simulink model "nmpc_sim"  (Simulink 8.8)
settings: Solver=ode45  StartTime=0.0  StopTime=20  RelTol=1e-3  EnableMultiTasking=on
InitFcn:
  | clear;close all;clc;
  | 
  | a=[-0.1832;558;118.45;9.6154e+03;...
  |     1.3712;5.1011e+03;641;426;6557;7.34;4484;0.016];
  | k=1;
  | x5d=50;
  | 
  | Ts=1e-4;
  | 
  | du=0.005;
StopFcn:
  | for i=1:4
  |     X(1:length(Measurements.signals(i).values(:,2)),i)=Measurements.signals(i).values(:,2);
  |     Xd(1:length(Measurements.signals(i).values(:,1)),i)=Measurements.signals(i).values(:,1);
  | end
  | 
  | U=Control.signals(2).values;
  | Ud=Control.signals(1).values;
  | 
  | Tnmpc=tnmpc.signals(1).values;
  | 
  | save exp_data X Xd U Ud Tnmpc;
values from neighbouring files (symbols this model uses):
  tnmpc = telapse/Ns    [nmpc_acado.m]
  ud = u(9)    [nmpc_acado.m]
undefined symbols (not defined in the file or in its folder): xd
settings Model: Creator=TIEUPHI  LastModifiedBy=trinhvv-admin
settings DataIOCC: SaveFormat=StructureWithTime  SignalLoggingSaveFormat=Dataset
settings DebuggingCC: UnderspecifiedInitializationDetection=Simplified  MergeDetectMultiDrivingBlocksExec=error  AllowSymbolicDim=off  StateNameClashWarn=none
settings HardwareCC: ProdBitPerPointer=64  ProdLargestAtomicFloat=Float  ProdIntDivRoundTo=Zero  ProdEndianess=LittleEndian  ProdHWDeviceType=Specified
settings GRTTargetCC: GeneratePreprocessorConditionals=Use local settings  CombineOutputUpdateFcns=on  GRTInterface=off

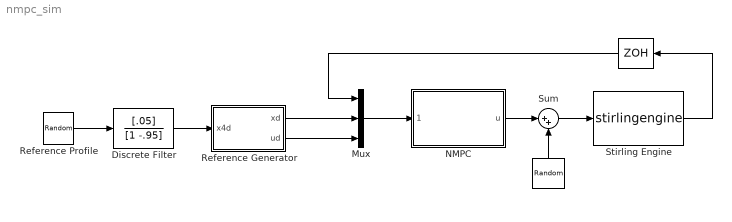
== system nmpc_sim ==
  "  " : ZeroOrderHold  SampleTime=Ts
  "   " : UniformRandomNumber  Minimum=-du  Maximum=du  Seed=1  SampleTime=Ts
  Discrete Filter : DiscreteFilter  Numerator=[.05]  Denominator=[1 -.95]  InitialStates=10.08*20  SampleTime=Ts
  Mux : Mux  Inputs=3
  NMPC : Subsystem
  Reference Generator : Subsystem
      mask init:
      | load ref_gen;
  Reference Profile : UniformRandomNumber  Minimum=7  Maximum=13  Seed=1234531  SampleTime=.5
  Stirling Engine : S-Function  InitFcn=try, set_param(gcb,'FunctionName','stirlingengine'), end  FunctionName=stirlingengine  Parameters=a,k,x5d  SFunctionModules=stirlingengine_wrapper  WizardData=DataTag0  SFunctionDeploymentMode=off  EnableBusSupport=off  mask(S-Function Builder){}
      mask help: Simulink:masks:SFunctionBuilder_MD
      mask init:
      | val = [[.9  0.75 0.75 1 1 .9 .9 1]',[1 1 0.75 0.75 .9 .9 1 .9]'];try , sys = get_param(gcb,'SfunBuilderFcnName');if isempty(sys), sys = get_param(gcb,'FunctionName'); end,catch, sys = get_param(gcb,'FunctionName'); end
      settings: CopyFcn=set_param(gcbh,'LinkStatus','none')  PreSaveFcn=try, set_param(gcb,'FunctionName','stirlingengine'), end  OpenFcn=sfunctionwizard(gcbh)
      mask Display: plot(val(:,1),val(:,2)),disp(sys), port_label('input',1,'u'), port_label('output',1,'y')
  Sum : Sum  Inputs=|++
  wires:
  Reference Generator/2(ud) -> Mux/3
  Reference Generator/1(xd) -> Mux/2
  Mux/1 -> NMPC/1(" ")
  Stirling Engine/1 -> "  "/1
  "  "/1 -> Mux/1
  Discrete Filter/1 -> Reference Generator/1(x4d)
  Reference Profile/1 -> Discrete Filter/1
  "   "/1 -> Sum/2
  NMPC/1(u) -> Sum/1
  Sum/1 -> Stirling Engine/1

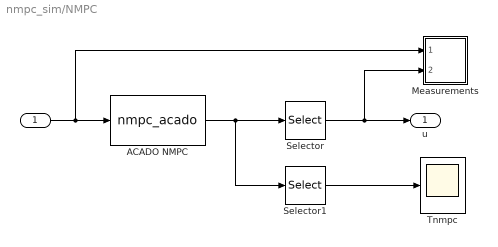
== system nmpc_sim/NMPC ==
  " " : Inport
  ACADO NMPC : MATLABFcn  MATLABFcn=nmpc_acado  OutputDimensions=2  OutputSignalType=real  SampleTime=Ts
  Measurements : Subsystem
  Selector : Selector  IndexOptions=Index vector (dialog)  Indices=1  OutputSizes=1
  Selector1 : Selector  IndexOptions=Index vector (dialog)  Indices=2  OutputSizes=1
  Tnmpc : Scope
  u : Outport
  wires:
  " "/1 -> Measurements/1(" "), ACADO NMPC/1
  ACADO NMPC/1 -> Selector1/1, Selector/1
  Selector/1 -> Measurements/2("   "), u/1
  Selector1/1 -> Tnmpc/1

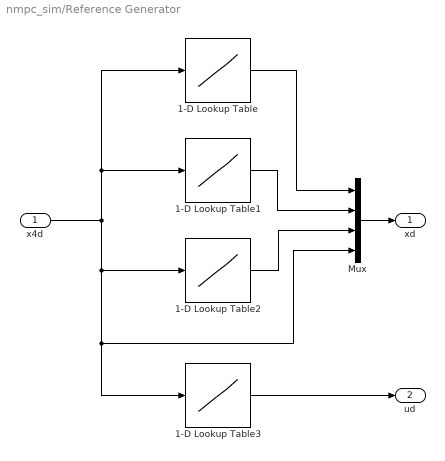
== system nmpc_sim/Reference Generator ==
  x4d : Inport
  1-D Lookup Table : Lookup_n-D  NumberOfTableDimensions=1  BreakpointsForDimension1=xd(:,4)  Table=xd(:,1)  RndMeth=Simplest  InputSameDT=on
  1-D Lookup Table1 : Lookup_n-D  NumberOfTableDimensions=1  BreakpointsForDimension1=xd(:,4)  Table=xd(:,2)  RndMeth=Simplest  InputSameDT=on
  1-D Lookup Table2 : Lookup_n-D  NumberOfTableDimensions=1  BreakpointsForDimension1=xd(:,4)  Table=xd(:,3)  RndMeth=Simplest  InputSameDT=on
  1-D Lookup Table3 : Lookup_n-D  NumberOfTableDimensions=1  BreakpointsForDimension1=xd(:,4)  Table=ud  RndMeth=Simplest  InputSameDT=on
  Mux : Mux
  xd : Outport
  ud : Outport  Port=2
  wires:
  x4d/1 -> Mux/4, 1-D Lookup Table3/1, 1-D Lookup Table2/1, 1-D Lookup Table1/1, 1-D Lookup Table/1
  Mux/1 -> xd/1
  1-D Lookup Table/1 -> Mux/1
  1-D Lookup Table1/1 -> Mux/2
  1-D Lookup Table2/1 -> Mux/3
  1-D Lookup Table3/1 -> ud/1

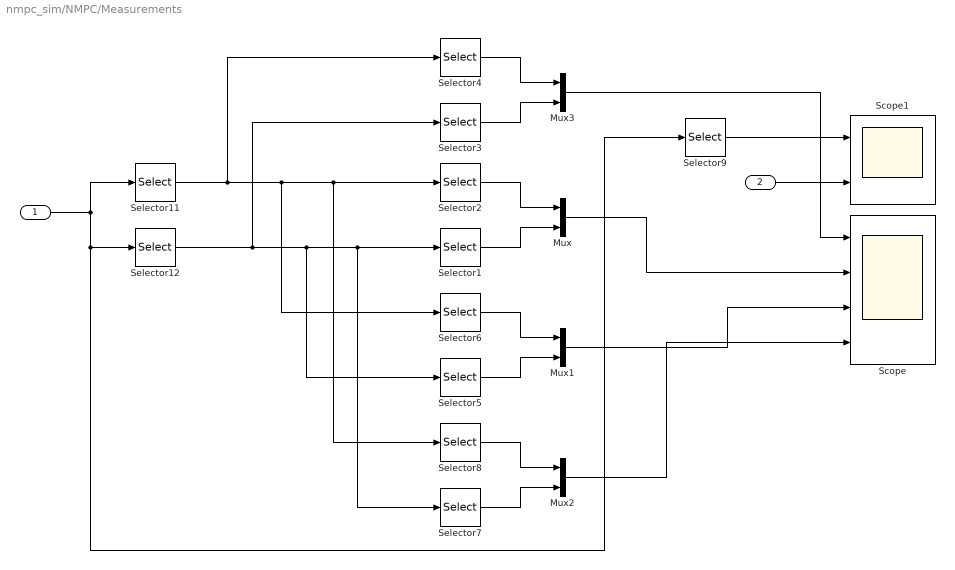
== system nmpc_sim/NMPC/Measurements ==
  " " : Inport
  "   " : Inport  Port=2
  Mux{,1..3} (4 alike) : Mux  Inputs=2
  Scope : Scope  NumInputPorts=4
  Scope1 : Scope  NumInputPorts=2
  Selector1 : Selector  InputPortWidth=4  IndexOptions=Index vector (dialog)  Indices=2  OutputSizes=1
  Selector11 : Selector  InputPortWidth=9  IndexOptions=Index vector (dialog)  Indices=[5:8]  OutputSizes=1
  Selector12 : Selector  InputPortWidth=9  IndexOptions=Index vector (dialog)  Indices=[1:4]  OutputSizes=1
  Selector2 : Selector  InputPortWidth=4  IndexOptions=Index vector (dialog)  Indices=2  OutputSizes=1
  Selector3 : Selector  InputPortWidth=4  IndexOptions=Index vector (dialog)  Indices=1  OutputSizes=1
  Selector4 : Selector  InputPortWidth=4  IndexOptions=Index vector (dialog)  Indices=1  OutputSizes=1
  Selector5 : Selector  InputPortWidth=4  IndexOptions=Index vector (dialog)  Indices=3  OutputSizes=1
  Selector6 : Selector  InputPortWidth=4  IndexOptions=Index vector (dialog)  Indices=3  OutputSizes=1
  Selector7 : Selector  InputPortWidth=4  IndexOptions=Index vector (dialog)  Indices=4  OutputSizes=1
  Selector8 : Selector  InputPortWidth=4  IndexOptions=Index vector (dialog)  Indices=4  OutputSizes=1
  Selector9 : Selector  InputPortWidth=9  IndexOptions=Index vector (dialog)  Indices=9  OutputSizes=1
  wires:
  Selector1/1 -> Mux/2
  Selector2/1 -> Mux/1
  Selector12/1 -> Selector3/1, Selector5/1, Selector7/1, Selector1/1
  Selector11/1 -> Selector6/1, Selector8/1, Selector2/1, Selector4/1
  Selector5/1 -> Mux1/2
  Selector6/1 -> Mux1/1
  Selector7/1 -> Mux2/2
  Selector8/1 -> Mux2/1
  Selector3/1 -> Mux3/2
  Selector4/1 -> Mux3/1
  " "/1 -> Selector11/1, Selector12/1, Selector9/1
  Mux3/1 -> Scope/1
  Mux/1 -> Scope/2
  Mux1/1 -> Scope/3
  Mux2/1 -> Scope/4
  Selector9/1 -> Scope1/1
  "   "/1 -> Scope1/2
